simulink model "comunicacion_arduno_2018"  (R2018a)
settings: Solver=VariableStepAuto  StartTime=0.0  StopTime=inf  RelTol=1e-3
undefined symbols (not defined in the file): LF, serial
libraries: instrumentlib x3, svdutilitieslib x1
settings Model: Creator=dcasta25  LastModifiedBy=dcasta25
settings DataIOCC: ReturnWorkspaceOutputs=on
settings DebuggingCC: UnconnectedInputMsg=none  UnconnectedOutputMsg=none  UnconnectedLineMsg=none
settings ModelReferenceCC: EnableRefExpFcnMdlSchedulingChecks=off
settings SFSimCC: SimUseLocalCustomCode=on
settings RTWCC: Description=Generic Real-Time Target  RTWUseLocalCustomCode=on

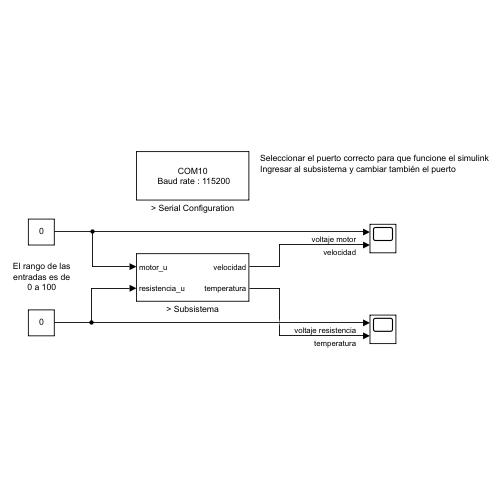
[thumbnail: Simulink's stored preview of the top-level diagram]
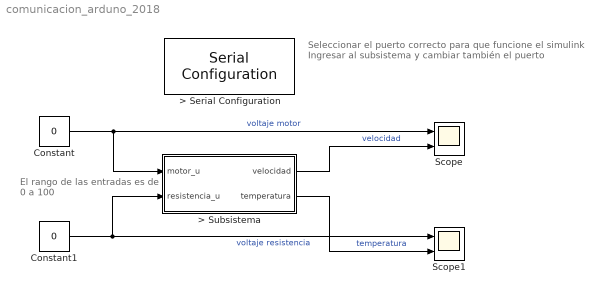
== system comunicacion_arduno_2018 ==
  note: El rango de las entradas es de 0 a 100
  note: Seleccionar el puerto correcto para que funcione el simulink
      | Ingresar al subsistema y cambiar también el puerto
  > Serial Configuration : instrumentlib/Serial Configuration  Priority=-200000  ObjConstructor=serial('COM10');  ComPortMenu=COM10  ComPort=COM10  BaudRate=115200  DataBits=8  Parity=none  StopBits=1  ByteOrder=LittleEndian  FlowControl=none  Timeout=10
  > Subsistema : Subsystem
      mask Display: image('CapturaDePantalla2023_11_14070130.png')
  Constant : Constant  Value=0
  Constant1 : Constant  Value=0
  Scope : Scope  NumInputPorts=2
  Scope1 : Scope  NumInputPorts=2
  wires:
  > Subsistema/1(velocidad) -> Scope/2  "velocidad"
  Constant/1 -> > Subsistema/1(motor_u), Scope/1  "voltaje motor"
  Constant1/1 -> Scope1/1, > Subsistema/2(resistencia_u)  "voltaje resistencia"
  > Subsistema/2(temperatura) -> Scope1/2  "temperatura"

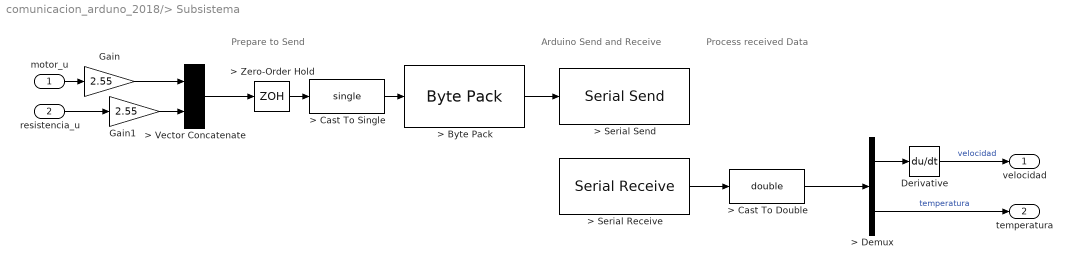
== system comunicacion_arduno_2018/> Subsistema ==
  note: Process received Data
  note: Arduino Send and Receive
  note: Prepare to Send
  motor_u : Inport
  resistencia_u : Inport  Port=2
  > Byte Pack : svdutilitieslib/Byte Pack  maskPackedDataType=uint32  datatypes={'single'}  byteAlign=4  blockPlatform=tic2000
  > Cast To Double : DataTypeConversion  OutDataTypeStr=double
  > Cast To Single : DataTypeConversion  OutDataTypeStr=single
  > Demux : Demux  Outputs=2
  > Serial Receive : instrumentlib/Serial Receive  Priority=1  ObjConstructor=serial('COM10');  ComPortMenu=COM10  ComPort=COM10  DataType=single  Header=A  Terminator=LF ('\n')  DataSize=[1 2]  EnableBlockingMode=on  ActionDataUnavailable=Output last received value  CustomValue=0  SampleTime=0.05
  > Serial Send : instrumentlib/Serial Send  Priority=1  ObjConstructor=serial('COM10');  ComPortMenu=COM10  ComPort=COM10  Terminator=<none>  EnableBlockingMode=on
  > Vector Concatenate : Concatenate
  > Zero-Order Hold : ZeroOrderHold  SampleTime=0.05
  Derivative : Derivative
  Gain : Gain  Gain=2.55
  Gain1 : Gain  Gain=2.55
  velocidad : Outport
  temperatura : Outport  Port=2
  wires:
  > Zero-Order Hold/1 -> > Cast To Single/1
  > Vector Concatenate/1 -> > Zero-Order Hold/1
  > Cast To Single/1 -> > Byte Pack/1
  > Cast To Double/1 -> > Demux/1
  > Byte Pack/1 -> > Serial Send/1
  resistencia_u/1 -> Gain1/1
  Derivative/1 -> velocidad/1  "velocidad"
  > Serial Receive/1 -> > Cast To Double/1
  > Demux/1 -> Derivative/1
  > Demux/2 -> temperatura/1  "temperatura"
  motor_u/1 -> Gain/1
  Gain/1 -> > Vector Concatenate/1
  Gain1/1 -> > Vector Concatenate/2
